simulink model "SegwaySim"  (R2023a)
settings: Solver=FixedStepAuto  StartTime=0.0  StopTime=10  FixedStep=1e-4  RelTol=1e-3
PreLoadFcn:
  | init
InitFcn:
  | ROBLabCONST
undefined symbols (not defined in the file or in its folder): Copycat, eta, K, Km, Kz, La, N, q_0, qdot_0, Ra, ref, Tm
settings Model: Creator=dervint  LastModifiedBy=dervint

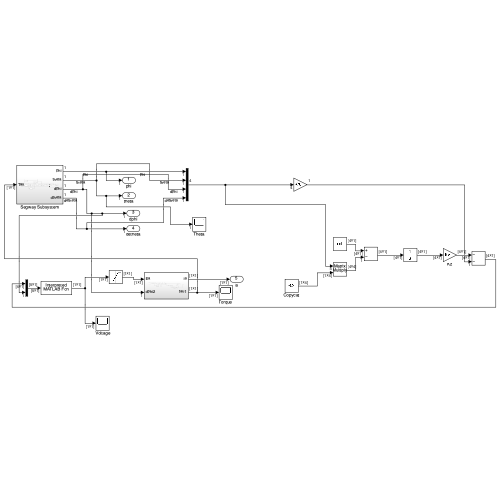
[thumbnail: Simulink's stored preview of the top-level diagram]
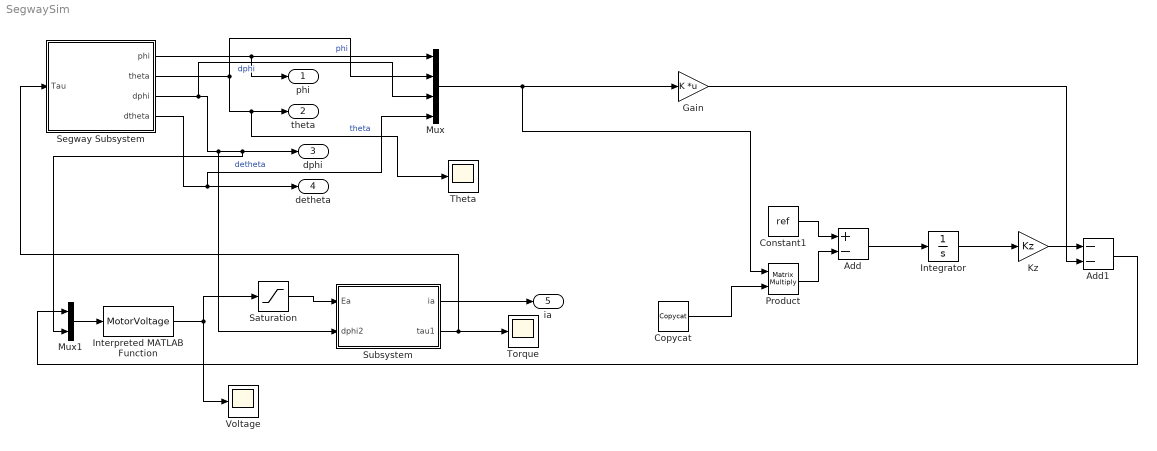
== system SegwaySim ==
  " Voltage" : Scope
  Add : Sum  Inputs=+-
  Add1 : Sum  Inputs=--
  Constant1 : Constant  Value=ref  VectorParams1D=off
  Copycat : Constant  Value=Copycat  VectorParams1D=off
  Gain : Gain  Gain=K  Multiplication=Matrix(K*u)
  Integrator : Integrator
  Interpreted MATLAB Function : MATLABFcn  MATLABFcn=MotorVoltage  Output1D=off
  Kz : Gain  Gain=Kz
  Mux : Mux
  Mux1 : Mux  Inputs=2
  Product : Product  Inputs=**  Multiplication=Matrix(*)
  Saturation : Saturate  UpperLimit=12  LowerLimit=0
  Segway Subsystem : Subsystem
  Subsystem : Subsystem
  Theta : Scope
  Torque : Scope
  phi : Outport
  theta : Outport  Port=2
  dphi : Outport  Port=3
  detheta : Outport  Port=4
  ia : Outport  Port=5
  wires:
  Segway Subsystem/1(phi) -> Mux/1, phi/1  "phi"
  Segway Subsystem/2(theta) -> Theta/1, theta/1, Mux/2  "theta"
  Segway Subsystem/3(dphi) -> Mux/3, dphi/1, Mux1/2, Subsystem/2(dphi2)  "dphi"
  Segway Subsystem/4(dtheta) -> Mux/4, detheta/1  "detheta"
  Mux/1 -> Product/1, Gain/1
  Subsystem/2(tau1) -> Torque/1, Segway Subsystem/1(Tau)
  Interpreted MATLAB Function/1 -> " Voltage"/1, Saturation/1
  Mux1/1 -> Interpreted MATLAB Function/1
  Subsystem/1(ia) -> ia/1
  Constant1/1 -> Add/1
  Add/1 -> Integrator/1
  Integrator/1 -> Kz/1
  Copycat/1 -> Product/2
  Product/1 -> Add/2
  Saturation/1 -> Subsystem/1(Ea)
  Kz/1 -> Add1/1
  Gain/1 -> Add1/2
  Add1/1 -> Mux1/1

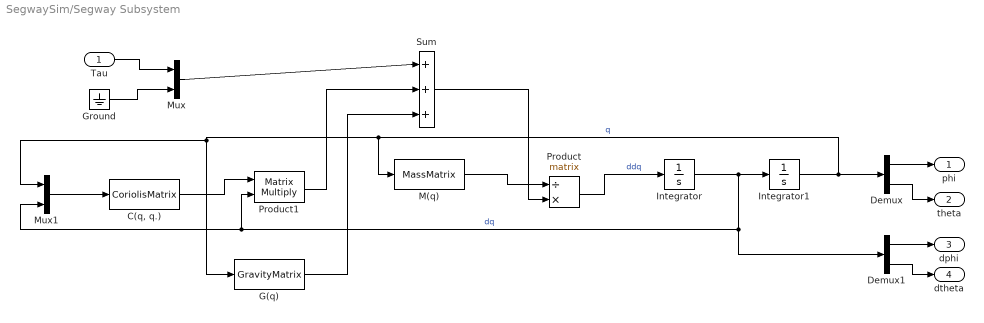
== system SegwaySim/Segway Subsystem ==
  Tau : Inport
  "C(q, q.)" : MATLABFcn  MATLABFcn=CoriolisMatrix  Output1D=off
  Demux : Demux  Outputs=2
  Demux1 : Demux  Outputs=2
  G(q) : MATLABFcn  MATLABFcn=GravityMatrix
  Ground : Ground
  Integrator : Integrator  InitialCondition=qdot_0
  Integrator1 : Integrator  InitialCondition=q_0
  M(q) : MATLABFcn  MATLABFcn=MassMatrix  Output1D=off
  Mux : Mux  Inputs=2
  Mux1 : Mux  Inputs=2
  Product : Product  Inputs=/*  Multiplication=Matrix(*)
  Product1 : Product  Multiplication=Matrix(*)
  Sum : Sum  Inputs=|+++
  phi : Outport
  theta : Outport  Port=2
  dphi : Outport  Port=3
  dtheta : Outport  Port=4
  wires:
  Tau/1 -> Mux/1
  Ground/1 -> Mux/2
  Mux/1 -> Sum/1
  Sum/1 -> Product/2
  Product/1 -> Integrator/1  "ddq"
  Integrator/1 -> Demux1/1, Product1/2, Mux1/2, Integrator1/1  "dq"
  Integrator1/1 -> M(q)/1, Mux1/1, G(q)/1, Demux/1  "q"
  Demux/1 -> phi/1
  Demux/2 -> theta/1
  Demux1/1 -> dphi/1
  Demux1/2 -> dtheta/1
  G(q)/1 -> Sum/3
  Mux1/1 -> "C(q, q.)"/1
  M(q)/1 -> Product/1
  "C(q, q.)"/1 -> Product1/1
  Product1/1 -> Sum/2

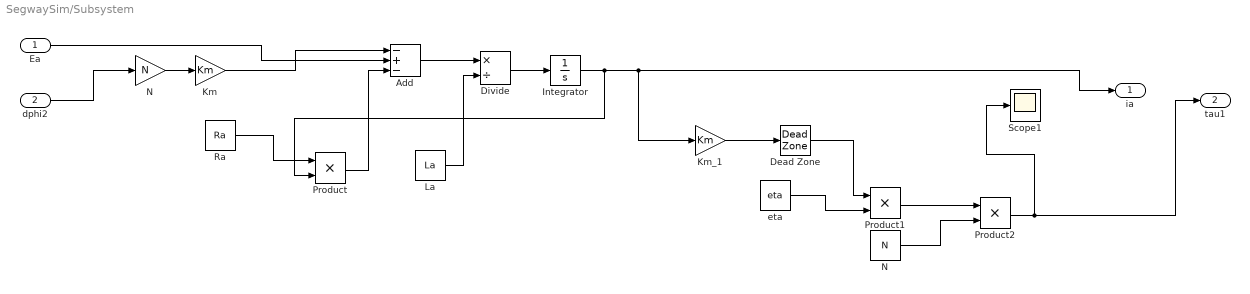
== system SegwaySim/Subsystem ==
  Ea : Inport
  dphi2 : Inport  Port=2
  Add : Sum  Inputs=-+-
  Dead Zone : DeadZone  LowerValue=-Tm  UpperValue=Tm
  Divide : Product  Inputs=*/
  Integrator : Integrator
  Km : Gain  Gain=Km
  Km_1 : Gain  Gain=Km
  La : Constant  Value=La
  N : Constant  Value=N
  "N " : Gain  Gain=N
  Product : Product
  Product1 : Product
  Product2 : Product
  Ra : Constant  Value=Ra
  Scope1 : Scope
  eta : Constant  Value=eta
  ia : Outport
  tau1 : Outport  Port=2
  wires:
  Integrator/1 -> ia/1, Km_1/1, Product/2
  Product2/1 -> tau1/1, Scope1/1
  Divide/1 -> Integrator/1
  Product1/1 -> Product2/1
  Add/1 -> Divide/1
  eta/1 -> Product1/2
  Dead Zone/1 -> Product1/1
  Km/1 -> Add/1
  Product/1 -> Add/3
  N/1 -> Product2/2
  Ea/1 -> Add/2
  Ra/1 -> Product/1
  "N "/1 -> Km/1
  Km_1/1 -> Dead Zone/1
  La/1 -> Divide/2
  dphi2/1 -> "N "/1
